simulink model "Fazy1"  (R2024b)
settings: Solver=VariableStepAuto  StartTime=0.0  StopTime=10.0  MaxStep=5  RelTol=1e-3
values from neighbouring files (symbols this model uses):
  bX = 1    [Lab5.m]
  czasskok = 500    [Lab5.m]    (also in MocGrzalkiPI.m; PrawyCz1.m = 0; PrawyCz2.m; Spr2.m = 1000)
  W = 0.01    [Lab5.m]
  war1 = 0    [Lab5.m]
  war2 = dx / (W^2)    (= 10000)    [Lab5.m]
  X = 1    [Lab5.m]
settings Model: Creator=pawli  LastModifiedBy=pawli

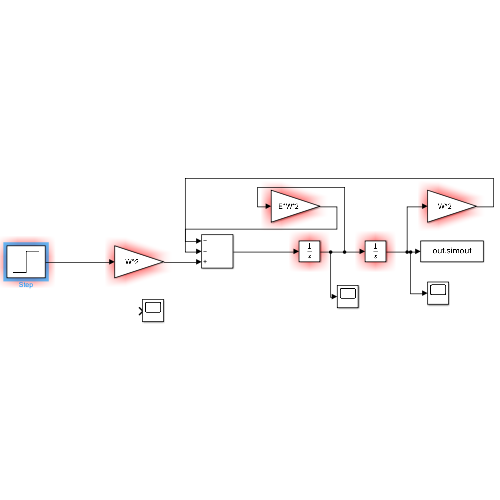
[thumbnail: Simulink's stored preview of the top-level diagram]
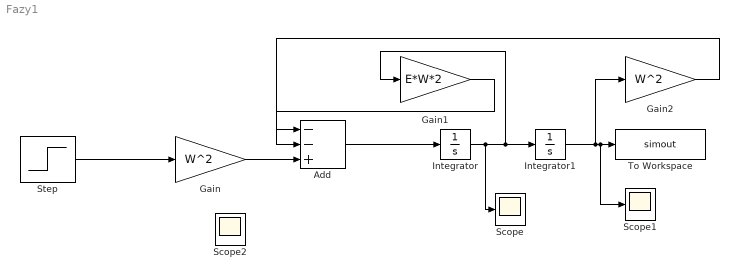
== system Fazy1 ==
  Add : Sum  Inputs=--+
  Gain : Gain  Gain=W^2
  Gain1 : Gain  Gain=E*W*2
  Gain2 : Gain  Gain=W^2
  Integrator : Integrator  InitialCondition=war1
  Integrator1 : Integrator  InitialCondition=war2
  Scope : Scope
  Scope1 : Scope
  Scope2 : Scope
  Step : Step  Time=czasskok  Before=X  After=X+bX  SampleTime=0
  To Workspace : ToWorkspace  VariableName=simout  SampleTime=-1
  wires:
  Gain/1 -> Add/3
  Add/1 -> Integrator/1
  Integrator/1 -> Scope/1, Gain1/1, Integrator1/1
  Gain1/1 -> Add/1
  Integrator1/1 -> Scope1/1, To Workspace/1, Gain2/1
  Gain2/1 -> Add/2
  Step/1 -> Gain/1
